simulink model "ScenarioManager1"  (R2024a)
settings: Solver=FixedStepDiscrete  StartTime=0.0  StopTime=10.0  FixedStep=0.1  RelTol=1e-3
values from neighbouring files (symbols this model uses):
  AIRCRAFT1_GOAL : value not decoded    [project_params.sldd]
  AIRCRAFT1_START : value not decoded    [project_params.sldd]
  AIRCRAFT2_GOAL : value not decoded    [project_params.sldd]
  AIRCRAFT2_START : value not decoded    [project_params.sldd]
settings Model: DataDictionary=project_params.sldd  Creator=amir  LastModifiedBy=amir
settings SolverCC: ZeroCrossControl=DisableAll  EnableFixedStepZeroCrossing=on
settings DataIOCC: SaveOutput=off  SaveTime=off
settings GRTTargetCC: CombineOutputUpdateFcns=off  MatFileLogging=off

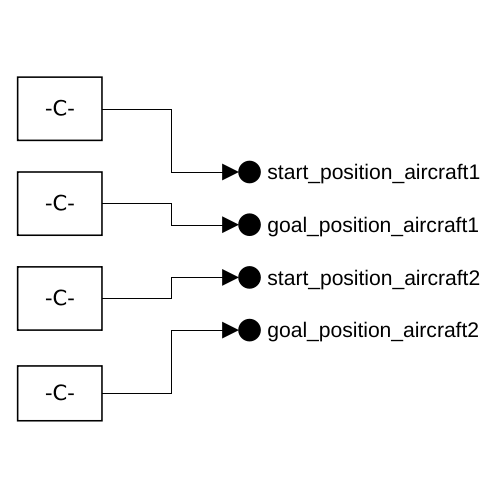
[thumbnail: Simulink's stored preview of the top-level diagram]
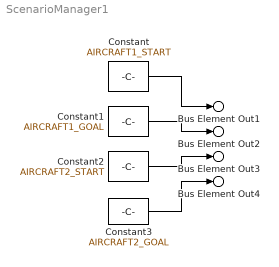
== system ScenarioManager1 ==
  Constant : Constant  Value=AIRCRAFT1_START
  Constant1 : Constant  Value=AIRCRAFT1_GOAL
  Constant2 : Constant  Value=AIRCRAFT2_START
  Constant3 : Constant  Value=AIRCRAFT2_GOAL
  Bus Element Out1 : Outport  PortName=start_position_aircraft1
  Bus Element Out2 : Outport  Port=2  PortName=goal_position_aircraft1
  Bus Element Out3 : Outport  Port=3  PortName=start_position_aircraft2
  Bus Element Out4 : Outport  Port=4  PortName=goal_position_aircraft2
  wires:
  Constant/1 -> Bus Element Out1/1
  Constant1/1 -> Bus Element Out2/1
  Constant2/1 -> Bus Element Out3/1
  Constant3/1 -> Bus Element Out4/1
